simulink library "halout"  (R2021b)
settings: Solver=VariableStepAuto  StartTime=0.0  StopTime=10.0  RelTol=1e-3
undefined symbols (not defined in the file): C_TASK_5MS_S, FALSE, KHAL_CAN1TxReq_flg, KHAL_CAN2TxReq_flg, KHAL_CAN3FD3VCU1toNIDECTxReq_flg, KHAL_CAN3FD3VCU1TxReq_flg, KHAL_CAN3FD3VCU2E2E_flg, KHAL_CAN3FD3VCU2toNIDECE2E_flg, KHAL_CAN3FD3VCU2toNIDECTxReq_flg, KHAL_CAN3FD3VCU2TxReq_flg, KHAL_CAN3TxReq_flg, KHAL_CAN4FD4CE1000E2E_flg, KHAL_CAN4FD4CE1000TxReq_flg, KHAL_CAN4TxReq_flg, KHAL_CAN5TxReq_flg, KHAL_CAN7TxReq_flg, ONE_INT, TRUE, ZERO_INT
libraries: FVT_lib x258, simulink x115
(part 14 of 17)

== system halout/HAL_OUT/CAN3/FD3_VCU2_toNIDEC_0x154/RrTMTqReqtoNidec ==
  RrTMTqReqtoNidec : Inport
  Data Type Conversion : DataTypeConversion  OutDataTypeStr=uint16  RndMeth=Round
  convert_out : FVT_lib/hal/convert_out  gain=1  offset=-530
  CAN3_Rr_TMTqReq_toNidec : Outport
  wires:
  Data Type Conversion/1 -> CAN3_Rr_TMTqReq_toNidec/1
  convert_out/1 -> Data Type Conversion/1
  RrTMTqReqtoNidec/1 -> convert_out/1

== system halout/HAL_OUT/CAN3/FD3_VCU2_toNIDEC_0x154/RrTorqMaxtoNidec ==
  RrTorqMaxtoNidec : Inport
  Data Type Conversion : DataTypeConversion  OutDataTypeStr=uint16  RndMeth=Round
  CAN3_Rr_TorqMax_toNidec : Outport
  wires:
  Data Type Conversion/1 -> CAN3_Rr_TorqMax_toNidec/1
  RrTorqMaxtoNidec/1 -> Data Type Conversion/1

== system halout/HAL_OUT/CAN3/FD3_VCU2_toNIDEC_0x154/RrTorqMintoNidec ==
  RrTorqMintoNidec : Inport
  Data Type Conversion : DataTypeConversion  OutDataTypeStr=uint16  RndMeth=Round
  convert_out : FVT_lib/hal/convert_out  gain=1  offset=-1022
  CAN3_Rr_TorqMin_toNidec : Outport
  wires:
  Data Type Conversion/1 -> CAN3_Rr_TorqMin_toNidec/1
  convert_out/1 -> Data Type Conversion/1
  RrTorqMintoNidec/1 -> convert_out/1

== system halout/HAL_OUT/CAN3/FD3_VCU2_toNIDEC_0x154/RrUdcMaxtoNidec ==
  RrUdcMaxtoNidec : Inport
  Data Type Conversion : DataTypeConversion  OutDataTypeStr=uint16  RndMeth=Round
  CAN3_Rr_UdcMax_toNidec : Outport
  wires:
  Data Type Conversion/1 -> CAN3_Rr_UdcMax_toNidec/1
  RrUdcMaxtoNidec/1 -> Data Type Conversion/1

== system halout/HAL_OUT/CAN3/FD3_VCU2_toNIDEC_0x154/RrUdcMintoNidec ==
  RrUdcMintoNidec : Inport
  Data Type Conversion : DataTypeConversion  OutDataTypeStr=uint16  RndMeth=Round
  CAN3_Rr_UdcMin_toNidec : Outport
  wires:
  Data Type Conversion/1 -> CAN3_Rr_UdcMin_toNidec/1
  RrUdcMintoNidec/1 -> Data Type Conversion/1

== system halout/HAL_OUT/CAN3/FD3_VCU5_0x155/ActAPSPosn ==
  ActAPSPosn : Inport
  Data Type Conversion : DataTypeConversion  OutDataTypeStr=uint8  RndMeth=Round
  convert_out : FVT_lib/hal/convert_out  gain=0.394  offset=0
  CAN3_ActAPSPosn : Outport
  wires:
  Data Type Conversion/1 -> CAN3_ActAPSPosn/1
  convert_out/1 -> Data Type Conversion/1
  ActAPSPosn/1 -> convert_out/1

== system halout/HAL_OUT/CAN3/FD3_VCU5_0x155/FrEDUSpd ==
  FrEDUSpd : Inport
  Data Type Conversion : DataTypeConversion  OutDataTypeStr=uint16  RndMeth=Round
  convert_out : FVT_lib/hal/convert_out  gain=1  offset=-2000
  CAN3_Fr_EDUSpd : Outport
  wires:
  Data Type Conversion/1 -> CAN3_Fr_EDUSpd/1
  convert_out/1 -> Data Type Conversion/1
  FrEDUSpd/1 -> convert_out/1

== system halout/HAL_OUT/CAN3/FD3_VCU5_0x155/FrEDUSpdValid ==
  FrEDUSpdValid : Inport
  Data Type Conversion : DataTypeConversion  OutDataTypeStr=uint8  RndMeth=Round
  CAN3_Fr_EDUSpdValid : Outport
  wires:
  Data Type Conversion/1 -> CAN3_Fr_EDUSpdValid/1
  FrEDUSpdValid/1 -> Data Type Conversion/1

== system halout/HAL_OUT/CAN3/FD3_VCU5_0x155/RrEDUSpd ==
  RrEDUSpd : Inport
  Data Type Conversion : DataTypeConversion  OutDataTypeStr=uint16  RndMeth=Round
  convert_out : FVT_lib/hal/convert_out  gain=1  offset=-2000
  CAN3_Rr_EDUSpd : Outport
  wires:
  Data Type Conversion/1 -> CAN3_Rr_EDUSpd/1
  convert_out/1 -> Data Type Conversion/1
  RrEDUSpd/1 -> convert_out/1

== system halout/HAL_OUT/CAN3/FD3_VCU5_0x155/RrEDUSpdValid ==
  RrEDUSpdValid : Inport
  Data Type Conversion : DataTypeConversion  OutDataTypeStr=uint8  RndMeth=Round
  CAN3_Rr_EDUSpdValid : Outport
  wires:
  Data Type Conversion/1 -> CAN3_Rr_EDUSpdValid/1
  RrEDUSpdValid/1 -> Data Type Conversion/1

== system halout/HAL_OUT/CAN3/GW3_CE100_0_0x1C3/CrashOutputSts ==
  CrashOutputSts : Inport
  Data Type Conversion : DataTypeConversion  OutDataTypeStr=uint8  RndMeth=Round
  CAN3_CrashOutputSts : Outport
  wires:
  Data Type Conversion/1 -> CAN3_CrashOutputSts/1
  CrashOutputSts/1 -> Data Type Conversion/1

== system halout/HAL_OUT/CAN3/GW3_CE100_0_0x1C3/DriverSeatBeltCmd ==
  DriverSeatBeltCmd : Inport
  Data Type Conversion : DataTypeConversion  OutDataTypeStr=uint8  RndMeth=Round
  CAN3_DriverSeatBeltCmd : Outport
  wires:
  Data Type Conversion/1 -> CAN3_DriverSeatBeltCmd/1
  DriverSeatBeltCmd/1 -> Data Type Conversion/1

== system halout/HAL_OUT/CAN3/GW3_CE100_0_0x1C3/VehSpeed ==
  VehSpeed : Inport
  Data Type Conversion : DataTypeConversion  OutDataTypeStr=uint16  RndMeth=Round
  convert_out : FVT_lib/hal/convert_out  gain=0.125  offset=0
  CAN3_VehSpeed : Outport
  wires:
  Data Type Conversion/1 -> CAN3_VehSpeed/1
  convert_out/1 -> Data Type Conversion/1
  VehSpeed/1 -> convert_out/1

== system halout/HAL_OUT/CAN4/FD4_C100_0_0x202/FDCCHAEACEnDemandCmd ==
  FDCCHAEACEnDemandCmd : Inport
  Data Type Conversion : DataTypeConversion  OutDataTypeStr=uint8  RndMeth=Round
  CAN4_FDC_CHA_EACEnDemand_Cmd : Outport
  wires:
  Data Type Conversion/1 -> CAN4_FDC_CHA_EACEnDemand_Cmd/1
  FDCCHAEACEnDemandCmd/1 -> Data Type Conversion/1

== system halout/HAL_OUT/CAN4/FD4_CE100_0_0x116/APSStaSystem ==
  APSStaSystem : Inport
  Data Type Conversion : DataTypeConversion  OutDataTypeStr=uint8  RndMeth=Round
  CAN4_APS_Sta_System : Outport
  wires:
  Data Type Conversion/1 -> CAN4_APS_Sta_System/1
  APSStaSystem/1 -> Data Type Conversion/1

== system halout/HAL_OUT/CAN4/FD4_CE100_0_0x116/AllDoorSW ==
  AllDoorSW : Inport
  Data Type Conversion : DataTypeConversion  OutDataTypeStr=uint8  RndMeth=Round
  CAN4_AllDoorSW : Outport
  wires:
  Data Type Conversion/1 -> CAN4_AllDoorSW/1
  AllDoorSW/1 -> Data Type Conversion/1

== system halout/HAL_OUT/CAN4/FD4_CE100_0_0x116/AntiTheftSeatFold ==
  AntiTheftSeatFold : Inport
  Data Type Conversion : DataTypeConversion  OutDataTypeStr=uint8  RndMeth=Round
  CAN4_AntiTheftSeatFold : Outport
  wires:
  Data Type Conversion/1 -> CAN4_AntiTheftSeatFold/1
  AntiTheftSeatFold/1 -> Data Type Conversion/1

== system halout/HAL_OUT/CAN4/FD4_CE100_0_0x116/AntitheftSta ==
  AntitheftSta : Inport
  Data Type Conversion : DataTypeConversion  OutDataTypeStr=uint8  RndMeth=Round
  CAN4_AntitheftSta : Outport
  wires:
  Data Type Conversion/1 -> CAN4_AntitheftSta/1
  AntitheftSta/1 -> Data Type Conversion/1

== system halout/HAL_OUT/CAN4/FD4_CE100_0_0x116/BCMDoorLockSta ==
  BCMDoorLockSta : Inport
  Data Type Conversion : DataTypeConversion  OutDataTypeStr=uint8  RndMeth=Round
  CAN4_BCM_DoorLock_Sta : Outport
  wires:
  Data Type Conversion/1 -> CAN4_BCM_DoorLock_Sta/1
  BCMDoorLockSta/1 -> Data Type Conversion/1

== system halout/HAL_OUT/CAN4/FD4_CE100_0_0x116/BrakeLamp ==
  BrakeLamp : Inport
  Data Type Conversion : DataTypeConversion  OutDataTypeStr=uint8  RndMeth=Round
  CAN4_BrakeLamp : Outport
  wires:
  Data Type Conversion/1 -> CAN4_BrakeLamp/1
  BrakeLamp/1 -> Data Type Conversion/1

== system halout/HAL_OUT/CAN4/FD4_CE100_0_0x116/Byte_0 ==
  CS_VCU1_CAN4 : Inport
  BitwiseOR : simulink/Logic and Bit Operations/Bitwise Operator  logicop=OR  UseBitMask=off  BitMask=bin2dec('11011001')  BitMaskRealWorld=Stored Integer
  SignalPack : FVT_lib/hal/SignalPack  RightShiftCnt=0  BitMask=2^8-1  LeftShiftCnt=0
  UnitConverter : DataTypeConversion  OutDataTypeStr=uint8  RndMeth=Round
  UnitConverter1 : DataTypeConversion  OutDataTypeStr=uint8  RndMeth=Round
  Byte_0 : Outport
  wires:
  BitwiseOR/1 -> Byte_0/1
  UnitConverter/1 -> BitwiseOR/1
  SignalPack/1 -> UnitConverter/1
  UnitConverter1/1 -> SignalPack/1
  CS_VCU1_CAN4/1 -> UnitConverter1/1

== system halout/HAL_OUT/CAN4/FD4_CE100_0_0x116/Byte_1 ==
  RC_VCU1_CAN4 : Inport
  BitwiseOR : simulink/Logic and Bit Operations/Bitwise Operator  logicop=OR  UseBitMask=off  BitMask=bin2dec('11011001')  BitMaskRealWorld=Stored Integer
  SignalPack : FVT_lib/hal/SignalPack  RightShiftCnt=0  BitMask=2^4-1  LeftShiftCnt=0
  UnitConverter : DataTypeConversion  OutDataTypeStr=uint8  RndMeth=Round
  UnitConverter1 : DataTypeConversion  OutDataTypeStr=uint8  RndMeth=Round
  Byte_1 : Outport
  wires:
  BitwiseOR/1 -> Byte_1/1
  UnitConverter/1 -> BitwiseOR/1
  SignalPack/1 -> UnitConverter/1
  UnitConverter1/1 -> SignalPack/1
  RC_VCU1_CAN4/1 -> UnitConverter1/1

== system halout/HAL_OUT/CAN4/FD4_CE100_0_0x116/Byte_10 ==
  TimeSNDKCFbk : Inport
  BitwiseOR : simulink/Logic and Bit Operations/Bitwise Operator  logicop=OR  UseBitMask=off  BitMask=bin2dec('11011001')  BitMaskRealWorld=Stored Integer
  SignalPack : FVT_lib/hal/SignalPack  RightShiftCnt=8  BitMask=2^8-1  LeftShiftCnt=0
  UnitConverter : DataTypeConversion  OutDataTypeStr=uint8  RndMeth=Round
  UnitConverter1 : DataTypeConversion  OutDataTypeStr=uint32  RndMeth=Round
  Byte_10 : Outport
  wires:
  BitwiseOR/1 -> Byte_10/1
  UnitConverter/1 -> BitwiseOR/1
  SignalPack/1 -> UnitConverter/1
  UnitConverter1/1 -> SignalPack/1
  TimeSNDKCFbk/1 -> UnitConverter1/1

== system halout/HAL_OUT/CAN4/FD4_CE100_0_0x116/Byte_11 ==
  TimeSNDKCFbk : Inport
  BitwiseOR : simulink/Logic and Bit Operations/Bitwise Operator  logicop=OR  UseBitMask=off  BitMask=bin2dec('11011001')  BitMaskRealWorld=Stored Integer
  SignalPack : FVT_lib/hal/SignalPack  RightShiftCnt=0  BitMask=2^8-1  LeftShiftCnt=0
  UnitConverter : DataTypeConversion  OutDataTypeStr=uint8  RndMeth=Round
  UnitConverter1 : DataTypeConversion  OutDataTypeStr=uint32  RndMeth=Round
  Byte_11 : Outport
  wires:
  BitwiseOR/1 -> Byte_11/1
  UnitConverter/1 -> BitwiseOR/1
  SignalPack/1 -> UnitConverter/1
  UnitConverter1/1 -> SignalPack/1
  TimeSNDKCFbk/1 -> UnitConverter1/1

== system halout/HAL_OUT/CAN4/FD4_CE100_0_0x116/Byte_12 ==
  BCM_DoorLock_Sta : Inport
  DimmerEN : Inport  Port=2
  EquivAccPedalSWSta : Inport  Port=3
  HornCtrl : Inport  Port=4
  RoomLampH : Inport  Port=5
  RoomLampL : Inport  Port=6
  TailgateRemote : Inport  Port=7
  BitwiseOR : simulink/Logic and Bit Operations/Bitwise Operator  logicop=OR  UseBitMask=off  NumInputPorts=7  BitMask=bin2dec('11011001')  BitMaskRealWorld=Stored Integer
  SignalPack : FVT_lib/hal/SignalPack  RightShiftCnt=0  BitMask=2^1-1  LeftShiftCnt=5
  SignalPack1 : FVT_lib/hal/SignalPack  RightShiftCnt=0  BitMask=2^1-1  LeftShiftCnt=4
  SignalPack2 : FVT_lib/hal/SignalPack  RightShiftCnt=0  BitMask=2^1-1  LeftShiftCnt=7
  SignalPack3 : FVT_lib/hal/SignalPack  RightShiftCnt=0  BitMask=2^1-1  LeftShiftCnt=6
  SignalPack4 : FVT_lib/hal/SignalPack  RightShiftCnt=0  BitMask=2^1-1  LeftShiftCnt=3
  SignalPack5 : FVT_lib/hal/SignalPack  RightShiftCnt=0  BitMask=2^1-1  LeftShiftCnt=2
  SignalPack6 : FVT_lib/hal/SignalPack  RightShiftCnt=0  BitMask=2^2-1  LeftShiftCnt=0
  UnitConverter{,1..13} (14 alike) : DataTypeConversion  OutDataTypeStr=uint8  RndMeth=Round
  Byte_12 : Outport
  wires:
  BitwiseOR/1 -> Byte_12/1
  UnitConverter/1 -> BitwiseOR/1
  SignalPack/1 -> UnitConverter/1
  UnitConverter1/1 -> SignalPack/1
  BCM_DoorLock_Sta/1 -> UnitConverter1/1
  UnitConverter2/1 -> BitwiseOR/2
  SignalPack1/1 -> UnitConverter2/1
  UnitConverter3/1 -> SignalPack1/1
  DimmerEN/1 -> UnitConverter3/1
  UnitConverter4/1 -> BitwiseOR/3
  SignalPack2/1 -> UnitConverter4/1
  UnitConverter5/1 -> SignalPack2/1
  EquivAccPedalSWSta/1 -> UnitConverter5/1
  UnitConverter6/1 -> BitwiseOR/4
  SignalPack3/1 -> UnitConverter6/1
  UnitConverter7/1 -> SignalPack3/1
  HornCtrl/1 -> UnitConverter7/1
  UnitConverter8/1 -> BitwiseOR/5
  SignalPack4/1 -> UnitConverter8/1
  UnitConverter9/1 -> SignalPack4/1
  RoomLampH/1 -> UnitConverter9/1
  UnitConverter10/1 -> BitwiseOR/6
  SignalPack5/1 -> UnitConverter10/1
  UnitConverter11/1 -> SignalPack5/1
  RoomLampL/1 -> UnitConverter11/1
  UnitConverter12/1 -> BitwiseOR/7
  SignalPack6/1 -> UnitConverter12/1
  UnitConverter13/1 -> SignalPack6/1
  TailgateRemote/1 -> UnitConverter13/1

== system halout/HAL_OUT/CAN4/FD4_CE100_0_0x116/Byte_13 ==
  Dimmer : Inport
  BitwiseOR : simulink/Logic and Bit Operations/Bitwise Operator  logicop=OR  UseBitMask=off  BitMask=bin2dec('11011001')  BitMaskRealWorld=Stored Integer
  SignalPack : FVT_lib/hal/SignalPack  RightShiftCnt=0  BitMask=2^7-1  LeftShiftCnt=0
  UnitConverter : DataTypeConversion  OutDataTypeStr=uint8  RndMeth=Round
  UnitConverter1 : DataTypeConversion  OutDataTypeStr=uint8  RndMeth=Round
  Byte_13 : Outport
  wires:
  BitwiseOR/1 -> Byte_13/1
  UnitConverter/1 -> BitwiseOR/1
  SignalPack/1 -> UnitConverter/1
  UnitConverter1/1 -> SignalPack/1
  Dimmer/1 -> UnitConverter1/1

== system halout/HAL_OUT/CAN4/FD4_CE100_0_0x116/Byte_14 ==
  AntiTheftSeatFold : Inport
  AntitheftSta : Inport  Port=2
  CrashDetd : Inport  Port=3
  L_APM_WdwEnable : Inport  Port=4
  LockSetting : Inport  Port=5
  RTurnLP : Inport  Port=6
  BitwiseOR : simulink/Logic and Bit Operations/Bitwise Operator  logicop=OR  UseBitMask=off  NumInputPorts=6  BitMask=bin2dec('11011001')  BitMaskRealWorld=Stored Integer
  SignalPack : FVT_lib/hal/SignalPack  RightShiftCnt=0  BitMask=2^1-1  LeftShiftCnt=3
  SignalPack1 : FVT_lib/hal/SignalPack  RightShiftCnt=0  BitMask=2^2-1  LeftShiftCnt=1
  SignalPack2 : FVT_lib/hal/SignalPack  RightShiftCnt=0  BitMask=2^1-1  LeftShiftCnt=4
  SignalPack3 : FVT_lib/hal/SignalPack  RightShiftCnt=0  BitMask=2^1-1  LeftShiftCnt=5
  SignalPack4 : FVT_lib/hal/SignalPack  RightShiftCnt=0  BitMask=2^1-1  LeftShiftCnt=6
  SignalPack5 : FVT_lib/hal/SignalPack  RightShiftCnt=0  BitMask=2^1-1  LeftShiftCnt=0
  UnitConverter{,1..11} (12 alike) : DataTypeConversion  OutDataTypeStr=uint8  RndMeth=Round
  Byte_14 : Outport
  wires:
  BitwiseOR/1 -> Byte_14/1
  UnitConverter/1 -> BitwiseOR/1
  SignalPack/1 -> UnitConverter/1
  UnitConverter1/1 -> SignalPack/1
  AntiTheftSeatFold/1 -> UnitConverter1/1
  UnitConverter2/1 -> BitwiseOR/2
  SignalPack1/1 -> UnitConverter2/1
  UnitConverter3/1 -> SignalPack1/1
  AntitheftSta/1 -> UnitConverter3/1
  UnitConverter4/1 -> BitwiseOR/3
  SignalPack2/1 -> UnitConverter4/1
  UnitConverter5/1 -> SignalPack2/1
  CrashDetd/1 -> UnitConverter5/1
  UnitConverter6/1 -> BitwiseOR/4
  SignalPack3/1 -> UnitConverter6/1
  UnitConverter7/1 -> SignalPack3/1
  L_APM_WdwEnable/1 -> UnitConverter7/1
  UnitConverter8/1 -> BitwiseOR/5
  SignalPack4/1 -> UnitConverter8/1
  UnitConverter9/1 -> SignalPack4/1
  LockSetting/1 -> UnitConverter9/1
  UnitConverter10/1 -> BitwiseOR/6
  SignalPack5/1 -> UnitConverter10/1
  UnitConverter11/1 -> SignalPack5/1
  RTurnLP/1 -> UnitConverter11/1

== system halout/HAL_OUT/CAN4/FD4_CE100_0_0x116/Byte_15 ==
  BrakeLamp : Inport
  Fr_FogLamp : Inport  Port=2
  HazardSW : Inport  Port=3
  LBSD : Inport  Port=4
  LTurnLP : Inport  Port=5
  RBSD : Inport  Port=6
  ReverseLamp : Inport  Port=7
  Rr_FogLamp : Inport  Port=8
  BitwiseOR : simulink/Logic and Bit Operations/Bitwise Operator  logicop=OR  UseBitMask=off  NumInputPorts=8  BitMask=bin2dec('11011001')  BitMaskRealWorld=Stored Integer
  SignalPack : FVT_lib/hal/SignalPack  RightShiftCnt=0  BitMask=2^1-1  LeftShiftCnt=1
  SignalPack1 : FVT_lib/hal/SignalPack  RightShiftCnt=0  BitMask=2^1-1  LeftShiftCnt=4
  SignalPack2 : FVT_lib/hal/SignalPack  RightShiftCnt=0  BitMask=2^1-1  LeftShiftCnt=6
  SignalPack3 : FVT_lib/hal/SignalPack  RightShiftCnt=0  BitMask=2^1-1  LeftShiftCnt=2
  SignalPack4 : FVT_lib/hal/SignalPack  RightShiftCnt=0  BitMask=2^1-1  LeftShiftCnt=7
  SignalPack5 : FVT_lib/hal/SignalPack  RightShiftCnt=0  BitMask=2^1-1  LeftShiftCnt=3
  SignalPack6 : FVT_lib/hal/SignalPack  RightShiftCnt=0  BitMask=2^1-1  LeftShiftCnt=0
  SignalPack7 : FVT_lib/hal/SignalPack  RightShiftCnt=0  BitMask=2^1-1  LeftShiftCnt=5
  UnitConverter{,1..15} (16 alike) : DataTypeConversion  OutDataTypeStr=uint8  RndMeth=Round
  Byte_15 : Outport
  wires:
  BitwiseOR/1 -> Byte_15/1
  UnitConverter/1 -> BitwiseOR/1
  SignalPack/1 -> UnitConverter/1
  UnitConverter1/1 -> SignalPack/1
  BrakeLamp/1 -> UnitConverter1/1
  UnitConverter2/1 -> BitwiseOR/2
  SignalPack1/1 -> UnitConverter2/1
  UnitConverter3/1 -> SignalPack1/1
  Fr_FogLamp/1 -> UnitConverter3/1
  UnitConverter4/1 -> BitwiseOR/3
  SignalPack2/1 -> UnitConverter4/1
  UnitConverter5/1 -> SignalPack2/1
  HazardSW/1 -> UnitConverter5/1
  UnitConverter6/1 -> BitwiseOR/4
  SignalPack3/1 -> UnitConverter6/1
  UnitConverter7/1 -> SignalPack3/1
  LBSD/1 -> UnitConverter7/1
  UnitConverter8/1 -> BitwiseOR/5
  SignalPack4/1 -> UnitConverter8/1
  UnitConverter9/1 -> SignalPack4/1
  LTurnLP/1 -> UnitConverter9/1
  UnitConverter10/1 -> BitwiseOR/6
  SignalPack5/1 -> UnitConverter10/1
  UnitConverter11/1 -> SignalPack5/1
  RBSD/1 -> UnitConverter11/1
  UnitConverter12/1 -> BitwiseOR/7
  SignalPack6/1 -> UnitConverter12/1
  UnitConverter13/1 -> SignalPack6/1
  ReverseLamp/1 -> UnitConverter13/1
  UnitConverter14/1 -> BitwiseOR/8
  SignalPack7/1 -> UnitConverter14/1
  UnitConverter15/1 -> SignalPack7/1
  Rr_FogLamp/1 -> UnitConverter15/1

== system halout/HAL_OUT/CAN4/FD4_CE100_0_0x116/Byte_16 ==
  H_Beam : Inport
  LDRL : Inport  Port=2
  L_Beam : Inport  Port=3
  PosLamp : Inport  Port=4
  RDRL : Inport  Port=5
  WasherCtrl : Inport  Port=6
  WiperFixMode : Inport  Port=7
  BitwiseOR : simulink/Logic and Bit Operations/Bitwise Operator  logicop=OR  UseBitMask=off  NumInputPorts=7  BitMask=bin2dec('11011001')  BitMaskRealWorld=Stored Integer
  SignalPack : FVT_lib/hal/SignalPack  RightShiftCnt=0  BitMask=2^1-1  LeftShiftCnt=4
  SignalPack1 : FVT_lib/hal/SignalPack  RightShiftCnt=0  BitMask=2^1-1  LeftShiftCnt=6
  SignalPack2 : FVT_lib/hal/SignalPack  RightShiftCnt=0  BitMask=2^1-1  LeftShiftCnt=3
  SignalPack3 : FVT_lib/hal/SignalPack  RightShiftCnt=0  BitMask=2^1-1  LeftShiftCnt=5
  SignalPack4 : FVT_lib/hal/SignalPack  RightShiftCnt=0  BitMask=2^1-1  LeftShiftCnt=7
  SignalPack5 : FVT_lib/hal/SignalPack  RightShiftCnt=0  BitMask=2^2-1  LeftShiftCnt=1
  SignalPack6 : FVT_lib/hal/SignalPack  RightShiftCnt=0  BitMask=2^1-1  LeftShiftCnt=0
  UnitConverter{,1..13} (14 alike) : DataTypeConversion  OutDataTypeStr=uint8  RndMeth=Round
  Byte_16 : Outport
  wires:
  BitwiseOR/1 -> Byte_16/1
  UnitConverter/1 -> BitwiseOR/1
  SignalPack/1 -> UnitConverter/1
  UnitConverter1/1 -> SignalPack/1
  H_Beam/1 -> UnitConverter1/1
  UnitConverter2/1 -> BitwiseOR/2
  SignalPack1/1 -> UnitConverter2/1
  UnitConverter3/1 -> SignalPack1/1
  LDRL/1 -> UnitConverter3/1
  UnitConverter4/1 -> BitwiseOR/3
  SignalPack2/1 -> UnitConverter4/1
  UnitConverter5/1 -> SignalPack2/1
  L_Beam/1 -> UnitConverter5/1
  UnitConverter6/1 -> BitwiseOR/4
  SignalPack3/1 -> UnitConverter6/1
  UnitConverter7/1 -> SignalPack3/1
  PosLamp/1 -> UnitConverter7/1
  UnitConverter8/1 -> BitwiseOR/5
  SignalPack4/1 -> UnitConverter8/1
  UnitConverter9/1 -> SignalPack4/1
  RDRL/1 -> UnitConverter9/1
  UnitConverter10/1 -> BitwiseOR/6
  SignalPack5/1 -> UnitConverter10/1
  UnitConverter11/1 -> SignalPack5/1
  WasherCtrl/1 -> UnitConverter11/1
  UnitConverter12/1 -> BitwiseOR/7
  SignalPack6/1 -> UnitConverter12/1
  UnitConverter13/1 -> SignalPack6/1
  WiperFixMode/1 -> UnitConverter13/1

== system halout/HAL_OUT/CAN4/FD4_CE100_0_0x116/Byte_17 ==
  Fr_Wiper_H : Inport
  Fr_Wiper_L : Inport  Port=2
  MirrorCtrl : Inport  Port=3
  Rr_Defog : Inport  Port=4
  Rr_Wiper : Inport  Port=5
  TailgateHDSW : Inport  Port=6
  TrunkRel : Inport  Port=7
  BitwiseOR : simulink/Logic and Bit Operations/Bitwise Operator  logicop=OR  UseBitMask=off  NumInputPorts=7  BitMask=bin2dec('11011001')  BitMaskRealWorld=Stored Integer
  SignalPack : FVT_lib/hal/SignalPack  RightShiftCnt=0  BitMask=2^1-1  LeftShiftCnt=5
  SignalPack1 : FVT_lib/hal/SignalPack  RightShiftCnt=0  BitMask=2^1-1  LeftShiftCnt=6
  SignalPack2 : FVT_lib/hal/SignalPack  RightShiftCnt=0  BitMask=2^2-1  LeftShiftCnt=3
  SignalPack3 : FVT_lib/hal/SignalPack  RightShiftCnt=0  BitMask=2^1-1  LeftShiftCnt=0
  SignalPack4 : FVT_lib/hal/SignalPack  RightShiftCnt=0  BitMask=2^1-1  LeftShiftCnt=7
  SignalPack5 : FVT_lib/hal/SignalPack  RightShiftCnt=0  BitMask=2^1-1  LeftShiftCnt=2
  SignalPack6 : FVT_lib/hal/SignalPack  RightShiftCnt=0  BitMask=2^1-1  LeftShiftCnt=1
  UnitConverter{,1..13} (14 alike) : DataTypeConversion  OutDataTypeStr=uint8  RndMeth=Round
  Byte_17 : Outport
  wires:
  BitwiseOR/1 -> Byte_17/1
  UnitConverter/1 -> BitwiseOR/1
  SignalPack/1 -> UnitConverter/1
  UnitConverter1/1 -> SignalPack/1
  Fr_Wiper_H/1 -> UnitConverter1/1
  UnitConverter2/1 -> BitwiseOR/2
  SignalPack1/1 -> UnitConverter2/1
  UnitConverter3/1 -> SignalPack1/1
  Fr_Wiper_L/1 -> UnitConverter3/1
  UnitConverter4/1 -> BitwiseOR/3
  SignalPack2/1 -> UnitConverter4/1
  UnitConverter5/1 -> SignalPack2/1
  MirrorCtrl/1 -> UnitConverter5/1
  UnitConverter6/1 -> BitwiseOR/4
  SignalPack3/1 -> UnitConverter6/1
  UnitConverter7/1 -> SignalPack3/1
  Rr_Defog/1 -> UnitConverter7/1
  UnitConverter8/1 -> BitwiseOR/5
  SignalPack4/1 -> UnitConverter8/1
  UnitConverter9/1 -> SignalPack4/1
  Rr_Wiper/1 -> UnitConverter9/1
  UnitConverter10/1 -> BitwiseOR/6
  SignalPack5/1 -> UnitConverter10/1
  UnitConverter11/1 -> SignalPack5/1
  TailgateHDSW/1 -> UnitConverter11/1
  UnitConverter12/1 -> BitwiseOR/7
  SignalPack6/1 -> UnitConverter12/1
  UnitConverter13/1 -> SignalPack6/1
  TrunkRel/1 -> UnitConverter13/1

== system halout/HAL_OUT/CAN4/FD4_CE100_0_0x116/Byte_19 ==
  AllDoorSW : Inport
  DoorLockIND : Inport  Port=2
  Fr_ChargingDoorCtrl : Inport  Port=3
  HoodSW : Inport  Port=4
  PsDoorSW : Inport  Port=5
  RLDoorSW : Inport  Port=6
  RRDoorSW : Inport  Port=7
  BitwiseOR : simulink/Logic and Bit Operations/Bitwise Operator  logicop=OR  UseBitMask=off  NumInputPorts=7  BitMask=bin2dec('11011001')  BitMaskRealWorld=Stored Integer
  SignalPack : FVT_lib/hal/SignalPack  RightShiftCnt=0  BitMask=2^1-1  LeftShiftCnt=3
  SignalPack1 : FVT_lib/hal/SignalPack  RightShiftCnt=0  BitMask=2^1-1  LeftShiftCnt=4
  SignalPack2 : FVT_lib/hal/SignalPack  RightShiftCnt=0  BitMask=2^2-1  LeftShiftCnt=6
  SignalPack3 : FVT_lib/hal/SignalPack  RightShiftCnt=0  BitMask=2^1-1  LeftShiftCnt=5
  SignalPack4 : FVT_lib/hal/SignalPack  RightShiftCnt=0  BitMask=2^1-1  LeftShiftCnt=0
  SignalPack5 : FVT_lib/hal/SignalPack  RightShiftCnt=0  BitMask=2^1-1  LeftShiftCnt=1
  SignalPack6 : FVT_lib/hal/SignalPack  RightShiftCnt=0  BitMask=2^1-1  LeftShiftCnt=2
  UnitConverter{,1..13} (14 alike) : DataTypeConversion  OutDataTypeStr=uint8  RndMeth=Round
  Byte_19 : Outport
  wires:
  BitwiseOR/1 -> Byte_19/1
  UnitConverter/1 -> BitwiseOR/1
  SignalPack/1 -> UnitConverter/1
  UnitConverter1/1 -> SignalPack/1
  AllDoorSW/1 -> UnitConverter1/1
  UnitConverter2/1 -> BitwiseOR/2
  SignalPack1/1 -> UnitConverter2/1
  UnitConverter3/1 -> SignalPack1/1
  DoorLockIND/1 -> UnitConverter3/1
  UnitConverter4/1 -> BitwiseOR/3
  SignalPack2/1 -> UnitConverter4/1
  UnitConverter5/1 -> SignalPack2/1
  Fr_ChargingDoorCtrl/1 -> UnitConverter5/1
  UnitConverter6/1 -> BitwiseOR/4
  SignalPack3/1 -> UnitConverter6/1
  UnitConverter7/1 -> SignalPack3/1
  HoodSW/1 -> UnitConverter7/1
  UnitConverter8/1 -> BitwiseOR/5
  SignalPack4/1 -> UnitConverter8/1
  UnitConverter9/1 -> SignalPack4/1
  PsDoorSW/1 -> UnitConverter9/1
  UnitConverter10/1 -> BitwiseOR/6
  SignalPack5/1 -> UnitConverter10/1
  UnitConverter11/1 -> SignalPack5/1
  RLDoorSW/1 -> UnitConverter11/1
  UnitConverter12/1 -> BitwiseOR/7
  SignalPack6/1 -> UnitConverter12/1
  UnitConverter13/1 -> SignalPack6/1
  RRDoorSW/1 -> UnitConverter13/1

== system halout/HAL_OUT/CAN4/FD4_CE100_0_0x116/Byte_2 ==
  CC_Crl_Sta : Inport
  Dr_SeatSta : Inport  Port=2
  MSA_Crl_Sta : Inport  Port=3
  BitwiseOR : simulink/Logic and Bit Operations/Bitwise Operator  logicop=OR  UseBitMask=off  NumInputPorts=3  BitMask=bin2dec('11011001')  BitMaskRealWorld=Stored Integer
  SignalPack : FVT_lib/hal/SignalPack  RightShiftCnt=0  BitMask=2^3-1  LeftShiftCnt=0
  SignalPack1 : FVT_lib/hal/SignalPack  RightShiftCnt=0  BitMask=2^2-1  LeftShiftCnt=6
  SignalPack2 : FVT_lib/hal/SignalPack  RightShiftCnt=0  BitMask=2^3-1  LeftShiftCnt=3
  UnitConverter{,1..5} (6 alike) : DataTypeConversion  OutDataTypeStr=uint8  RndMeth=Round
  Byte_2 : Outport
  wires:
  BitwiseOR/1 -> Byte_2/1
  UnitConverter/1 -> BitwiseOR/1
  SignalPack/1 -> UnitConverter/1
  UnitConverter1/1 -> SignalPack/1
  CC_Crl_Sta/1 -> UnitConverter1/1
  UnitConverter2/1 -> BitwiseOR/2
  SignalPack1/1 -> UnitConverter2/1
  UnitConverter3/1 -> SignalPack1/1
  Dr_SeatSta/1 -> UnitConverter3/1
  UnitConverter4/1 -> BitwiseOR/3
  SignalPack2/1 -> UnitConverter4/1
  UnitConverter5/1 -> SignalPack2/1
  MSA_Crl_Sta/1 -> UnitConverter5/1

== system halout/HAL_OUT/CAN4/FD4_CE100_0_0x116/Byte_20 ==
  CTDCtrl : Inport
  FD_TBOX_VehData_Sta : Inport  Port=2
  Rr_ChargingDoorCtrl : Inport  Port=3
  BitwiseOR : simulink/Logic and Bit Operations/Bitwise Operator  logicop=OR  UseBitMask=off  NumInputPorts=3  BitMask=bin2dec('11011001')  BitMaskRealWorld=Stored Integer
  SignalPack : FVT_lib/hal/SignalPack  RightShiftCnt=0  BitMask=2^2-1  LeftShiftCnt=4
  SignalPack1 : FVT_lib/hal/SignalPack  RightShiftCnt=0  BitMask=2^4-1  LeftShiftCnt=0
  SignalPack2 : FVT_lib/hal/SignalPack  RightShiftCnt=0  BitMask=2^2-1  LeftShiftCnt=6
  UnitConverter{,1..5} (6 alike) : DataTypeConversion  OutDataTypeStr=uint8  RndMeth=Round
  Byte_20 : Outport
  wires:
  BitwiseOR/1 -> Byte_20/1
  UnitConverter/1 -> BitwiseOR/1
  SignalPack/1 -> UnitConverter/1
  UnitConverter1/1 -> SignalPack/1
  CTDCtrl/1 -> UnitConverter1/1
  UnitConverter2/1 -> BitwiseOR/2
  SignalPack1/1 -> UnitConverter2/1
  UnitConverter3/1 -> SignalPack1/1
  FD_TBOX_VehData_Sta/1 -> UnitConverter3/1
  UnitConverter4/1 -> BitwiseOR/3
  SignalPack2/1 -> UnitConverter4/1
  UnitConverter5/1 -> SignalPack2/1
  Rr_ChargingDoorCtrl/1 -> UnitConverter5/1

== system halout/HAL_OUT/CAN4/FD4_CE100_0_0x116/Byte_21 ==
  FD_DKC_VehData_Sta : Inport
  FD_TBOX_VehData_Err : Inport  Port=2
  BitwiseOR : simulink/Logic and Bit Operations/Bitwise Operator  logicop=OR  UseBitMask=off  NumInputPorts=2  BitMask=bin2dec('11011001')  BitMaskRealWorld=Stored Integer
  SignalPack : FVT_lib/hal/SignalPack  RightShiftCnt=0  BitMask=2^4-1  LeftShiftCnt=0
  SignalPack1 : FVT_lib/hal/SignalPack  RightShiftCnt=0  BitMask=2^4-1  LeftShiftCnt=4
  UnitConverter{,1..3} (4 alike) : DataTypeConversion  OutDataTypeStr=uint8  RndMeth=Round
  Byte_21 : Outport
  wires:
  BitwiseOR/1 -> Byte_21/1
  UnitConverter/1 -> BitwiseOR/1
  SignalPack/1 -> UnitConverter/1
  UnitConverter1/1 -> SignalPack/1
  FD_DKC_VehData_Sta/1 -> UnitConverter1/1
  UnitConverter2/1 -> BitwiseOR/2
  SignalPack1/1 -> UnitConverter2/1
  UnitConverter3/1 -> SignalPack1/1
  FD_TBOX_VehData_Err/1 -> UnitConverter3/1

== system halout/HAL_OUT/CAN4/FD4_CE100_0_0x116/Byte_22 ==
  FD_DKC_VehData_Err : Inport
  FD_TBOX_DTCData_Sta : Inport  Port=2
  BitwiseOR : simulink/Logic and Bit Operations/Bitwise Operator  logicop=OR  UseBitMask=off  NumInputPorts=2  BitMask=bin2dec('11011001')  BitMaskRealWorld=Stored Integer
  SignalPack : FVT_lib/hal/SignalPack  RightShiftCnt=0  BitMask=2^4-1  LeftShiftCnt=4
  SignalPack1 : FVT_lib/hal/SignalPack  RightShiftCnt=0  BitMask=2^4-1  LeftShiftCnt=0
  UnitConverter{,1..3} (4 alike) : DataTypeConversion  OutDataTypeStr=uint8  RndMeth=Round
  Byte_22 : Outport
  wires:
  BitwiseOR/1 -> Byte_22/1
  UnitConverter/1 -> BitwiseOR/1
  SignalPack/1 -> UnitConverter/1
  UnitConverter1/1 -> SignalPack/1
  FD_DKC_VehData_Err/1 -> UnitConverter1/1
  UnitConverter2/1 -> BitwiseOR/2
  SignalPack1/1 -> UnitConverter2/1
  UnitConverter3/1 -> SignalPack1/1
  FD_TBOX_DTCData_Sta/1 -> UnitConverter3/1

== system halout/HAL_OUT/CAN4/FD4_CE100_0_0x116/Byte_23 ==
  DKCAuthSta : Inport
  FD_TBOX_DTCData_Err : Inport  Port=2
  LampPwr : Inport  Port=3
  BitwiseOR : simulink/Logic and Bit Operations/Bitwise Operator  logicop=OR  UseBitMask=off  NumInputPorts=3  BitMask=bin2dec('11011001')  BitMaskRealWorld=Stored Integer
  SignalPack : FVT_lib/hal/SignalPack  RightShiftCnt=0  BitMask=2^2-1  LeftShiftCnt=0
  SignalPack1 : FVT_lib/hal/SignalPack  RightShiftCnt=0  BitMask=2^4-1  LeftShiftCnt=4
  SignalPack2 : FVT_lib/hal/SignalPack  RightShiftCnt=0  BitMask=2^1-1  LeftShiftCnt=3
  UnitConverter{,1..5} (6 alike) : DataTypeConversion  OutDataTypeStr=uint8  RndMeth=Round
  Byte_23 : Outport
  wires:
  BitwiseOR/1 -> Byte_23/1
  UnitConverter/1 -> BitwiseOR/1
  SignalPack/1 -> UnitConverter/1
  UnitConverter1/1 -> SignalPack/1
  DKCAuthSta/1 -> UnitConverter1/1
  UnitConverter2/1 -> BitwiseOR/2
  SignalPack1/1 -> UnitConverter2/1
  UnitConverter3/1 -> SignalPack1/1
  FD_TBOX_DTCData_Err/1 -> UnitConverter3/1
  UnitConverter4/1 -> BitwiseOR/3
  SignalPack2/1 -> UnitConverter4/1
  UnitConverter5/1 -> SignalPack2/1
  LampPwr/1 -> UnitConverter5/1

== system halout/HAL_OUT/CAN4/FD4_CE100_0_0x116/Byte_25 ==
  CtrlFrBMSCCUCIR : Inport
  CtrlFrEDUINVERTER : Inport  Port=2
  CtrlFrIRC1 : Inport  Port=3
  CtrlFrPwrStbA1P : Inport  Port=4
  DrDoorSW : Inport  Port=5
  HWResetSta : Inport  Port=6
  MirrorDefog : Inport  Port=7
  BitwiseOR : simulink/Logic and Bit Operations/Bitwise Operator  logicop=OR  UseBitMask=off  NumInputPorts=7  BitMask=bin2dec('11011001')  BitMaskRealWorld=Stored Integer
  SignalPack : FVT_lib/hal/SignalPack  RightShiftCnt=0  BitMask=2^1-1  LeftShiftCnt=0
  SignalPack1 : FVT_lib/hal/SignalPack  RightShiftCnt=0  BitMask=2^1-1  LeftShiftCnt=1
  SignalPack2 : FVT_lib/hal/SignalPack  RightShiftCnt=0  BitMask=2^1-1  LeftShiftCnt=2
  SignalPack3 : FVT_lib/hal/SignalPack  RightShiftCnt=0  BitMask=2^1-1  LeftShiftCnt=3
  SignalPack4 : FVT_lib/hal/SignalPack  RightShiftCnt=0  BitMask=2^1-1  LeftShiftCnt=6
  SignalPack5 : FVT_lib/hal/SignalPack  RightShiftCnt=0  BitMask=2^2-1  LeftShiftCnt=4
  SignalPack6 : FVT_lib/hal/SignalPack  RightShiftCnt=0  BitMask=2^1-1  LeftShiftCnt=7
  UnitConverter{,1..13} (14 alike) : DataTypeConversion  OutDataTypeStr=uint8  RndMeth=Round
  Byte_25 : Outport
  wires:
  BitwiseOR/1 -> Byte_25/1
  UnitConverter/1 -> BitwiseOR/1
  SignalPack/1 -> UnitConverter/1
  UnitConverter1/1 -> SignalPack/1
  CtrlFrBMSCCUCIR/1 -> UnitConverter1/1
  UnitConverter2/1 -> BitwiseOR/2
  SignalPack1/1 -> UnitConverter2/1
  UnitConverter3/1 -> SignalPack1/1
  CtrlFrEDUINVERTER/1 -> UnitConverter3/1
  UnitConverter4/1 -> BitwiseOR/3
  SignalPack2/1 -> UnitConverter4/1
  UnitConverter5/1 -> SignalPack2/1
  CtrlFrIRC1/1 -> UnitConverter5/1
  UnitConverter6/1 -> BitwiseOR/4
  SignalPack3/1 -> UnitConverter6/1
  UnitConverter7/1 -> SignalPack3/1
  CtrlFrPwrStbA1P/1 -> UnitConverter7/1
  UnitConverter8/1 -> BitwiseOR/5
  SignalPack4/1 -> UnitConverter8/1
  UnitConverter9/1 -> SignalPack4/1
  DrDoorSW/1 -> UnitConverter9/1
  UnitConverter10/1 -> BitwiseOR/6
  SignalPack5/1 -> UnitConverter10/1
  UnitConverter11/1 -> SignalPack5/1
  HWResetSta/1 -> UnitConverter11/1
  UnitConverter12/1 -> BitwiseOR/7
  SignalPack6/1 -> UnitConverter12/1
  UnitConverter13/1 -> SignalPack6/1
  MirrorDefog/1 -> UnitConverter13/1

== system halout/HAL_OUT/CAN4/FD4_CE100_0_0x116/Byte_26 ==
  APS_Sta_System : Inport
  CTDLockSW : Inport  Port=2
  CTDUnlockSW : Inport  Port=3
  BitwiseOR : simulink/Logic and Bit Operations/Bitwise Operator  logicop=OR  UseBitMask=off  NumInputPorts=3  BitMask=bin2dec('11011001')  BitMaskRealWorld=Stored Integer
  SignalPack : FVT_lib/hal/SignalPack  RightShiftCnt=0  BitMask=2^3-1  LeftShiftCnt=3
  SignalPack1 : FVT_lib/hal/SignalPack  RightShiftCnt=0  BitMask=2^1-1  LeftShiftCnt=7
  SignalPack2 : FVT_lib/hal/SignalPack  RightShiftCnt=0  BitMask=2^1-1  LeftShiftCnt=6
  UnitConverter{,1..5} (6 alike) : DataTypeConversion  OutDataTypeStr=uint8  RndMeth=Round
  Byte_26 : Outport
  wires:
  BitwiseOR/1 -> Byte_26/1
  UnitConverter/1 -> BitwiseOR/1
  SignalPack/1 -> UnitConverter/1
  UnitConverter1/1 -> SignalPack/1
  APS_Sta_System/1 -> UnitConverter1/1
  UnitConverter2/1 -> BitwiseOR/2
  SignalPack1/1 -> UnitConverter2/1
  UnitConverter3/1 -> SignalPack1/1
  CTDLockSW/1 -> UnitConverter3/1
  UnitConverter4/1 -> BitwiseOR/3
  SignalPack2/1 -> UnitConverter4/1
  UnitConverter5/1 -> SignalPack2/1
  CTDUnlockSW/1 -> UnitConverter5/1

== system halout/HAL_OUT/CAN4/FD4_CE100_0_0x116/Byte_27 ==
  CtrlDrPwrStbA2 : Inport
  Tailgate_SW : Inport  Port=2
  BitwiseOR : simulink/Logic and Bit Operations/Bitwise Operator  logicop=OR  UseBitMask=off  NumInputPorts=2  BitMask=bin2dec('11011001')  BitMaskRealWorld=Stored Integer
  SignalPack : FVT_lib/hal/SignalPack  RightShiftCnt=0  BitMask=2^1-1  LeftShiftCnt=6
  SignalPack1 : FVT_lib/hal/SignalPack  RightShiftCnt=0  BitMask=2^1-1  LeftShiftCnt=7
  UnitConverter{,1..3} (4 alike) : DataTypeConversion  OutDataTypeStr=uint8  RndMeth=Round
  Byte_27 : Outport
  wires:
  BitwiseOR/1 -> Byte_27/1
  UnitConverter/1 -> BitwiseOR/1
  SignalPack/1 -> UnitConverter/1
  UnitConverter1/1 -> SignalPack/1
  CtrlDrPwrStbA2/1 -> UnitConverter1/1
  UnitConverter2/1 -> BitwiseOR/2
  SignalPack1/1 -> UnitConverter2/1
  UnitConverter3/1 -> SignalPack1/1
  Tailgate_SW/1 -> UnitConverter3/1

== system halout/HAL_OUT/CAN4/FD4_CE100_0_0x116/Byte_3 ==
  H_Beam_ADB : Inport
  PwrSta : Inport  Port=2
  ReBrakeLPReq : Inport  Port=3
  ShiftGearPosn : Inport  Port=4
  BitwiseOR : simulink/Logic and Bit Operations/Bitwise Operator  logicop=OR  UseBitMask=off  NumInputPorts=4  BitMask=bin2dec('11011001')  BitMaskRealWorld=Stored Integer
  SignalPack : FVT_lib/hal/SignalPack  RightShiftCnt=0  BitMask=2^1-1  LeftShiftCnt=0
  SignalPack1 : FVT_lib/hal/SignalPack  RightShiftCnt=0  BitMask=2^3-1  LeftShiftCnt=2
  SignalPack2 : FVT_lib/hal/SignalPack  RightShiftCnt=0  BitMask=2^1-1  LeftShiftCnt=1
  SignalPack3 : FVT_lib/hal/SignalPack  RightShiftCnt=0  BitMask=2^3-1  LeftShiftCnt=5
  UnitConverter{,1..7} (8 alike) : DataTypeConversion  OutDataTypeStr=uint8  RndMeth=Round
  Byte_3 : Outport
  wires:
  BitwiseOR/1 -> Byte_3/1
  UnitConverter/1 -> BitwiseOR/1
  SignalPack/1 -> UnitConverter/1
  UnitConverter1/1 -> SignalPack/1
  H_Beam_ADB/1 -> UnitConverter1/1
  UnitConverter2/1 -> BitwiseOR/2
  SignalPack1/1 -> UnitConverter2/1
  UnitConverter3/1 -> SignalPack1/1
  PwrSta/1 -> UnitConverter3/1
  UnitConverter4/1 -> BitwiseOR/3
  SignalPack2/1 -> UnitConverter4/1
  UnitConverter5/1 -> SignalPack2/1
  ReBrakeLPReq/1 -> UnitConverter5/1
  UnitConverter6/1 -> BitwiseOR/4
  SignalPack3/1 -> UnitConverter6/1
  UnitConverter7/1 -> SignalPack3/1
  ShiftGearPosn/1 -> UnitConverter7/1

== system halout/HAL_OUT/CAN4/FD4_CE100_0_0x116/Byte_4 ==
  DKCTimeSN : Inport
  BitwiseOR : simulink/Logic and Bit Operations/Bitwise Operator  logicop=OR  UseBitMask=off  BitMask=bin2dec('11011001')  BitMaskRealWorld=Stored Integer
  SignalPack : FVT_lib/hal/SignalPack  RightShiftCnt=24  BitMask=2^8-1  LeftShiftCnt=0
  UnitConverter : DataTypeConversion  OutDataTypeStr=uint8  RndMeth=Round
  UnitConverter1 : DataTypeConversion  OutDataTypeStr=uint32  RndMeth=Round
  Byte_4 : Outport
  wires:
  BitwiseOR/1 -> Byte_4/1
  UnitConverter/1 -> BitwiseOR/1
  SignalPack/1 -> UnitConverter/1
  UnitConverter1/1 -> SignalPack/1
  DKCTimeSN/1 -> UnitConverter1/1

== system halout/HAL_OUT/CAN4/FD4_CE100_0_0x116/Byte_5 ==
  DKCTimeSN : Inport
  BitwiseOR : simulink/Logic and Bit Operations/Bitwise Operator  logicop=OR  UseBitMask=off  BitMask=bin2dec('11011001')  BitMaskRealWorld=Stored Integer
  SignalPack : FVT_lib/hal/SignalPack  RightShiftCnt=16  BitMask=2^8-1  LeftShiftCnt=0
  UnitConverter : DataTypeConversion  OutDataTypeStr=uint8  RndMeth=Round
  UnitConverter1 : DataTypeConversion  OutDataTypeStr=uint32  RndMeth=Round
  Byte_5 : Outport
  wires:
  BitwiseOR/1 -> Byte_5/1
  UnitConverter/1 -> BitwiseOR/1
  SignalPack/1 -> UnitConverter/1
  UnitConverter1/1 -> SignalPack/1
  DKCTimeSN/1 -> UnitConverter1/1

== system halout/HAL_OUT/CAN4/FD4_CE100_0_0x116/Byte_6 ==
  DKCTimeSN : Inport
  BitwiseOR : simulink/Logic and Bit Operations/Bitwise Operator  logicop=OR  UseBitMask=off  BitMask=bin2dec('11011001')  BitMaskRealWorld=Stored Integer
  SignalPack : FVT_lib/hal/SignalPack  RightShiftCnt=8  BitMask=2^8-1  LeftShiftCnt=0
  UnitConverter : DataTypeConversion  OutDataTypeStr=uint8  RndMeth=Round
  UnitConverter1 : DataTypeConversion  OutDataTypeStr=uint32  RndMeth=Round
  Byte_6 : Outport
  wires:
  BitwiseOR/1 -> Byte_6/1
  UnitConverter/1 -> BitwiseOR/1
  SignalPack/1 -> UnitConverter/1
  UnitConverter1/1 -> SignalPack/1
  DKCTimeSN/1 -> UnitConverter1/1

== system halout/HAL_OUT/CAN4/FD4_CE100_0_0x116/Byte_7 ==
  DKCTimeSN : Inport
  BitwiseOR : simulink/Logic and Bit Operations/Bitwise Operator  logicop=OR  UseBitMask=off  BitMask=bin2dec('11011001')  BitMaskRealWorld=Stored Integer
  SignalPack : FVT_lib/hal/SignalPack  RightShiftCnt=0  BitMask=2^8-1  LeftShiftCnt=0
  UnitConverter : DataTypeConversion  OutDataTypeStr=uint8  RndMeth=Round
  UnitConverter1 : DataTypeConversion  OutDataTypeStr=uint32  RndMeth=Round
  Byte_7 : Outport
  wires:
  BitwiseOR/1 -> Byte_7/1
  UnitConverter/1 -> BitwiseOR/1
  SignalPack/1 -> UnitConverter/1
  UnitConverter1/1 -> SignalPack/1
  DKCTimeSN/1 -> UnitConverter1/1

== system halout/HAL_OUT/CAN4/FD4_CE100_0_0x116/Byte_8 ==
  TimeSNDKCFbk : Inport
  BitwiseOR : simulink/Logic and Bit Operations/Bitwise Operator  logicop=OR  UseBitMask=off  BitMask=bin2dec('11011001')  BitMaskRealWorld=Stored Integer
  SignalPack : FVT_lib/hal/SignalPack  RightShiftCnt=24  BitMask=2^8-1  LeftShiftCnt=0
  UnitConverter : DataTypeConversion  OutDataTypeStr=uint8  RndMeth=Round
  UnitConverter1 : DataTypeConversion  OutDataTypeStr=uint32  RndMeth=Round
  Byte_8 : Outport
  wires:
  BitwiseOR/1 -> Byte_8/1
  UnitConverter/1 -> BitwiseOR/1
  SignalPack/1 -> UnitConverter/1
  UnitConverter1/1 -> SignalPack/1
  TimeSNDKCFbk/1 -> UnitConverter1/1

== system halout/HAL_OUT/CAN4/FD4_CE100_0_0x116/Byte_9 ==
  TimeSNDKCFbk : Inport
  BitwiseOR : simulink/Logic and Bit Operations/Bitwise Operator  logicop=OR  UseBitMask=off  BitMask=bin2dec('11011001')  BitMaskRealWorld=Stored Integer
  SignalPack : FVT_lib/hal/SignalPack  RightShiftCnt=16  BitMask=2^8-1  LeftShiftCnt=0
  UnitConverter : DataTypeConversion  OutDataTypeStr=uint8  RndMeth=Round
  UnitConverter1 : DataTypeConversion  OutDataTypeStr=uint32  RndMeth=Round
  Byte_9 : Outport
  wires:
  BitwiseOR/1 -> Byte_9/1
  UnitConverter/1 -> BitwiseOR/1
  SignalPack/1 -> UnitConverter/1
  UnitConverter1/1 -> SignalPack/1
  TimeSNDKCFbk/1 -> UnitConverter1/1

== system halout/HAL_OUT/CAN4/FD4_CE100_0_0x116/CCCrlSta ==
  CCCrlSta : Inport
  Data Type Conversion : DataTypeConversion  OutDataTypeStr=uint8  RndMeth=Round
  CAN4_CC_Crl_Sta : Outport
  wires:
  Data Type Conversion/1 -> CAN4_CC_Crl_Sta/1
  CCCrlSta/1 -> Data Type Conversion/1

== system halout/HAL_OUT/CAN4/FD4_CE100_0_0x116/CRC8_IfAction_Tx ==
  CAN_E2E_flg : Inport
  DataID1 : Inport  Port=2
  DataID2 : Inport  Port=3
  RawData : Inport  Port=4
  Data Type Conversion : DataTypeConversion  OutDataTypeStr=uint8
  If : If
  If Action Subsystem : Subsystem  TreatAsAtomicUnit=on
  If Action Subsystem1 : Subsystem  TreatAsAtomicUnit=on
  Merge : Merge
  CRC8 : Outport
  wires:
  If/2 -> If Action Subsystem/Action
  If/1 -> If Action Subsystem1/Action
  CAN_E2E_flg/1 -> [CAN_E2E_flg]
  DataID1/1 -> [DataID1]
  DataID2/1 -> [DataID2]
  RawData/1 -> [RawData]
  [CAN_E2E_flg] -> Data Type Conversion/1
  [DataID1] -> If Action Subsystem1/1(CAN_E2E_ID1)
  [DataID2] -> If Action Subsystem1/2(CAN_E2E_ID2)
  [RawData] -> If Action Subsystem1/3(Byte1)
  [RawData] -> If Action Subsystem/1(Byte1)
  If Action Subsystem1/1(CRC8_E2EResult) -> Merge/1
  If Action Subsystem/1(CRC8_Result) -> Merge/2
  Merge/1 -> CRC8/1
  Data Type Conversion/1 -> If/1

== system halout/HAL_OUT/CAN4/FD4_CE100_0_0x116/CSVCU1CAN4 ==
  CSVCU1CAN4 : Inport
  Data Type Conversion : DataTypeConversion  OutDataTypeStr=uint8  RndMeth=Round
  CAN4_CS_VCU1_CAN4 : Outport
  wires:
  Data Type Conversion/1 -> CAN4_CS_VCU1_CAN4/1
  CSVCU1CAN4/1 -> Data Type Conversion/1

== system halout/HAL_OUT/CAN4/FD4_CE100_0_0x116/CTDCtrl ==
  CTDCtrl : Inport
  Data Type Conversion : DataTypeConversion  OutDataTypeStr=uint8  RndMeth=Round
  CAN4_CTDCtrl : Outport
  wires:
  Data Type Conversion/1 -> CAN4_CTDCtrl/1
  CTDCtrl/1 -> Data Type Conversion/1

== system halout/HAL_OUT/CAN4/FD4_CE100_0_0x116/CTDLockSW ==
  CTDLockSW : Inport
  Data Type Conversion : DataTypeConversion  OutDataTypeStr=uint8  RndMeth=Round
  CAN4_CTDLockSW : Outport
  wires:
  Data Type Conversion/1 -> CAN4_CTDLockSW/1
  CTDLockSW/1 -> Data Type Conversion/1

== system halout/HAL_OUT/CAN4/FD4_CE100_0_0x116/CTDUnlockSW ==
  CTDUnlockSW : Inport
  Data Type Conversion : DataTypeConversion  OutDataTypeStr=uint8  RndMeth=Round
  CAN4_CTDUnlockSW : Outport
  wires:
  Data Type Conversion/1 -> CAN4_CTDUnlockSW/1
  CTDUnlockSW/1 -> Data Type Conversion/1

== system halout/HAL_OUT/CAN4/FD4_CE100_0_0x116/CrashDetd ==
  CrashDetd : Inport
  Data Type Conversion : DataTypeConversion  OutDataTypeStr=uint8  RndMeth=Round
  CAN4_CrashDetd : Outport
  wires:
  Data Type Conversion/1 -> CAN4_CrashDetd/1
  CrashDetd/1 -> Data Type Conversion/1

== system halout/HAL_OUT/CAN4/FD4_CE100_0_0x116/CtrlDrPwrStbA2 ==
  CtrlDrPwrStbA2 : Inport
  Data Type Conversion : DataTypeConversion  OutDataTypeStr=uint8  RndMeth=Round
  CAN4_CtrlDrPwrStbA2 : Outport
  wires:
  Data Type Conversion/1 -> CAN4_CtrlDrPwrStbA2/1
  CtrlDrPwrStbA2/1 -> Data Type Conversion/1

== system halout/HAL_OUT/CAN4/FD4_CE100_0_0x116/CtrlFrBMSCCUCIR ==
  CtrlFrBMSCCUCIR : Inport
  Data Type Conversion : DataTypeConversion  OutDataTypeStr=uint8  RndMeth=Round
  CAN4_CtrlFrBMSCCUCIR : Outport
  wires:
  Data Type Conversion/1 -> CAN4_CtrlFrBMSCCUCIR/1
  CtrlFrBMSCCUCIR/1 -> Data Type Conversion/1

== system halout/HAL_OUT/CAN4/FD4_CE100_0_0x116/CtrlFrEDUINVERTER ==
  CtrlFrEDUINVERTER : Inport
  Data Type Conversion : DataTypeConversion  OutDataTypeStr=uint8  RndMeth=Round
  CAN4_CtrlFrEDUINVERTER : Outport
  wires:
  Data Type Conversion/1 -> CAN4_CtrlFrEDUINVERTER/1
  CtrlFrEDUINVERTER/1 -> Data Type Conversion/1

== system halout/HAL_OUT/CAN4/FD4_CE100_0_0x116/CtrlFrIRC1 ==
  CtrlFrIRC1 : Inport
  Data Type Conversion : DataTypeConversion  OutDataTypeStr=uint8  RndMeth=Round
  CAN4_CtrlFrIRC1 : Outport
  wires:
  Data Type Conversion/1 -> CAN4_CtrlFrIRC1/1
  CtrlFrIRC1/1 -> Data Type Conversion/1

== system halout/HAL_OUT/CAN4/FD4_CE100_0_0x116/CtrlFrPwrStbA1P ==
  CtrlFrPwrStbA1P : Inport
  Data Type Conversion : DataTypeConversion  OutDataTypeStr=uint8  RndMeth=Round
  CAN4_CtrlFrPwrStbA1P : Outport
  wires:
  Data Type Conversion/1 -> CAN4_CtrlFrPwrStbA1P/1
  CtrlFrPwrStbA1P/1 -> Data Type Conversion/1

== system halout/HAL_OUT/CAN4/FD4_CE100_0_0x116/DKCAuthSta ==
  DKCAuthSta : Inport
  Data Type Conversion : DataTypeConversion  OutDataTypeStr=uint8  RndMeth=Round
  CAN4_DKCAuthSta : Outport
  wires:
  Data Type Conversion/1 -> CAN4_DKCAuthSta/1
  DKCAuthSta/1 -> Data Type Conversion/1

== system halout/HAL_OUT/CAN4/FD4_CE100_0_0x116/DKCTimeSN ==
  DKCTimeSN : Inport
  Data Type Conversion : DataTypeConversion  OutDataTypeStr=uint32  RndMeth=Round
  CAN4_DKCTimeSN : Outport
  wires:
  Data Type Conversion/1 -> CAN4_DKCTimeSN/1
  DKCTimeSN/1 -> Data Type Conversion/1

== system halout/HAL_OUT/CAN4/FD4_CE100_0_0x116/Dimmer ==
  Dimmer : Inport
  Data Type Conversion : DataTypeConversion  OutDataTypeStr=uint8  RndMeth=Round
  CAN4_Dimmer : Outport
  wires:
  Data Type Conversion/1 -> CAN4_Dimmer/1
  Dimmer/1 -> Data Type Conversion/1

== system halout/HAL_OUT/CAN4/FD4_CE100_0_0x116/DimmerEN ==
  DimmerEN : Inport
  Data Type Conversion : DataTypeConversion  OutDataTypeStr=uint8  RndMeth=Round
  CAN4_DimmerEN : Outport
  wires:
  Data Type Conversion/1 -> CAN4_DimmerEN/1
  DimmerEN/1 -> Data Type Conversion/1

== system halout/HAL_OUT/CAN4/FD4_CE100_0_0x116/DoorLockIND ==
  DoorLockIND : Inport
  Data Type Conversion : DataTypeConversion  OutDataTypeStr=uint8  RndMeth=Round
  CAN4_DoorLockIND : Outport
  wires:
  Data Type Conversion/1 -> CAN4_DoorLockIND/1
  DoorLockIND/1 -> Data Type Conversion/1

== system halout/HAL_OUT/CAN4/FD4_CE100_0_0x116/DrDoorSW ==
  DrDoorSW : Inport
  Data Type Conversion : DataTypeConversion  OutDataTypeStr=uint8  RndMeth=Round
  CAN4_DrDoorSW : Outport
  wires:
  Data Type Conversion/1 -> CAN4_DrDoorSW/1
  DrDoorSW/1 -> Data Type Conversion/1

== system halout/HAL_OUT/CAN4/FD4_CE100_0_0x116/DrSeatSta ==
  DrSeatSta : Inport
  Data Type Conversion : DataTypeConversion  OutDataTypeStr=uint8  RndMeth=Round
  CAN4_Dr_SeatSta : Outport
  wires:
  Data Type Conversion/1 -> CAN4_Dr_SeatSta/1
  DrSeatSta/1 -> Data Type Conversion/1

== system halout/HAL_OUT/CAN4/FD4_CE100_0_0x116/EquivAccPedalSWSta ==
  EquivAccPedalSWSta : Inport
  Data Type Conversion : DataTypeConversion  OutDataTypeStr=uint8  RndMeth=Round
  CAN4_EquivAccPedalSWSta : Outport
  wires:
  Data Type Conversion/1 -> CAN4_EquivAccPedalSWSta/1
  EquivAccPedalSWSta/1 -> Data Type Conversion/1

== system halout/HAL_OUT/CAN4/FD4_CE100_0_0x116/FDDKCVehDataErr ==
  FDDKCVehDataErr : Inport
  Data Type Conversion : DataTypeConversion  OutDataTypeStr=uint8  RndMeth=Round
  CAN4_FD_DKC_VehData_Err : Outport
  wires:
  Data Type Conversion/1 -> CAN4_FD_DKC_VehData_Err/1
  FDDKCVehDataErr/1 -> Data Type Conversion/1

== system halout/HAL_OUT/CAN4/FD4_CE100_0_0x116/FDDKCVehDataSta ==
  FDDKCVehDataSta : Inport
  Data Type Conversion : DataTypeConversion  OutDataTypeStr=uint8  RndMeth=Round
  CAN4_FD_DKC_VehData_Sta : Outport
  wires:
  Data Type Conversion/1 -> CAN4_FD_DKC_VehData_Sta/1
  FDDKCVehDataSta/1 -> Data Type Conversion/1

== system halout/HAL_OUT/CAN4/FD4_CE100_0_0x116/FDTBOXDTCDataErr ==
  FDTBOXDTCDataErr : Inport
  Data Type Conversion : DataTypeConversion  OutDataTypeStr=uint8  RndMeth=Round
  CAN4_FD_TBOX_DTCData_Err : Outport
  wires:
  Data Type Conversion/1 -> CAN4_FD_TBOX_DTCData_Err/1
  FDTBOXDTCDataErr/1 -> Data Type Conversion/1

== system halout/HAL_OUT/CAN4/FD4_CE100_0_0x116/FDTBOXDTCDataSta ==
  FDTBOXDTCDataSta : Inport
  Data Type Conversion : DataTypeConversion  OutDataTypeStr=uint8  RndMeth=Round
  CAN4_FD_TBOX_DTCData_Sta : Outport
  wires:
  Data Type Conversion/1 -> CAN4_FD_TBOX_DTCData_Sta/1
  FDTBOXDTCDataSta/1 -> Data Type Conversion/1

== system halout/HAL_OUT/CAN4/FD4_CE100_0_0x116/FDTBOXVehDataErr ==
  FDTBOXVehDataErr : Inport
  Data Type Conversion : DataTypeConversion  OutDataTypeStr=uint8  RndMeth=Round
  CAN4_FD_TBOX_VehData_Err : Outport
  wires:
  Data Type Conversion/1 -> CAN4_FD_TBOX_VehData_Err/1
  FDTBOXVehDataErr/1 -> Data Type Conversion/1

== system halout/HAL_OUT/CAN4/FD4_CE100_0_0x116/FDTBOXVehDataSta ==
  FDTBOXVehDataSta : Inport
  Data Type Conversion : DataTypeConversion  OutDataTypeStr=uint8  RndMeth=Round
  CAN4_FD_TBOX_VehData_Sta : Outport
  wires:
  Data Type Conversion/1 -> CAN4_FD_TBOX_VehData_Sta/1
  FDTBOXVehDataSta/1 -> Data Type Conversion/1

== system halout/HAL_OUT/CAN4/FD4_CE100_0_0x116/FrChargingDoorCtrl ==
  FrChargingDoorCtrl : Inport
  Data Type Conversion : DataTypeConversion  OutDataTypeStr=uint8  RndMeth=Round
  CAN4_Fr_ChargingDoorCtrl : Outport
  wires:
  Data Type Conversion/1 -> CAN4_Fr_ChargingDoorCtrl/1
  FrChargingDoorCtrl/1 -> Data Type Conversion/1

== system halout/HAL_OUT/CAN4/FD4_CE100_0_0x116/FrFogLamp ==
  FrFogLamp : Inport
  Data Type Conversion : DataTypeConversion  OutDataTypeStr=uint8  RndMeth=Round
  CAN4_Fr_FogLamp : Outport
  wires:
  Data Type Conversion/1 -> CAN4_Fr_FogLamp/1
  FrFogLamp/1 -> Data Type Conversion/1

== system halout/HAL_OUT/CAN4/FD4_CE100_0_0x116/FrWiperH ==
  FrWiperH : Inport
  Data Type Conversion : DataTypeConversion  OutDataTypeStr=uint8  RndMeth=Round
  CAN4_Fr_Wiper_H : Outport
  wires:
  Data Type Conversion/1 -> CAN4_Fr_Wiper_H/1
  FrWiperH/1 -> Data Type Conversion/1

== system halout/HAL_OUT/CAN4/FD4_CE100_0_0x116/FrWiperL ==
  FrWiperL : Inport
  Data Type Conversion : DataTypeConversion  OutDataTypeStr=uint8  RndMeth=Round
  CAN4_Fr_Wiper_L : Outport
  wires:
  Data Type Conversion/1 -> CAN4_Fr_Wiper_L/1
  FrWiperL/1 -> Data Type Conversion/1

== system halout/HAL_OUT/CAN4/FD4_CE100_0_0x116/HBeam ==
  HBeam : Inport
  Data Type Conversion : DataTypeConversion  OutDataTypeStr=uint8  RndMeth=Round
  CAN4_H_Beam : Outport
  wires:
  Data Type Conversion/1 -> CAN4_H_Beam/1
  HBeam/1 -> Data Type Conversion/1

== system halout/HAL_OUT/CAN4/FD4_CE100_0_0x116/HBeamADB ==
  HBeamADB : Inport
  Data Type Conversion : DataTypeConversion  OutDataTypeStr=uint8  RndMeth=Round
  CAN4_H_Beam_ADB : Outport
  wires:
  Data Type Conversion/1 -> CAN4_H_Beam_ADB/1
  HBeamADB/1 -> Data Type Conversion/1

== system halout/HAL_OUT/CAN4/FD4_CE100_0_0x116/HWResetSta ==
  HWResetSta : Inport
  Data Type Conversion : DataTypeConversion  OutDataTypeStr=uint8  RndMeth=Round
  CAN4_HWResetSta : Outport
  wires:
  Data Type Conversion/1 -> CAN4_HWResetSta/1
  HWResetSta/1 -> Data Type Conversion/1

== system halout/HAL_OUT/CAN4/FD4_CE100_0_0x116/HazardSW ==
  HazardSW : Inport
  Data Type Conversion : DataTypeConversion  OutDataTypeStr=uint8  RndMeth=Round
  CAN4_HazardSW : Outport
  wires:
  Data Type Conversion/1 -> CAN4_HazardSW/1
  HazardSW/1 -> Data Type Conversion/1

== system halout/HAL_OUT/CAN4/FD4_CE100_0_0x116/HoodSW ==
  HoodSW : Inport
  Data Type Conversion : DataTypeConversion  OutDataTypeStr=uint8  RndMeth=Round
  CAN4_HoodSW : Outport
  wires:
  Data Type Conversion/1 -> CAN4_HoodSW/1
  HoodSW/1 -> Data Type Conversion/1
